simulink model "timertest"  (R2019a)
settings: Solver=VariableStepAuto  StartTime=0.0  StopTime=3600 * 24 * 60  RelTol=1e-3
undefined symbols (not defined in the file or in its folder): f
libraries: instrumentlib x2
settings Model: Creator=brandt  LastModifiedBy=brandt

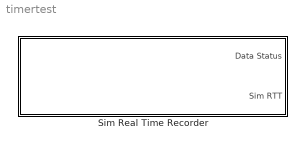
== system timertest ==
  Sim Real Time Recorder : Subsystem  AncestorBlock=gasLibrary/Sim Real Time Recorder

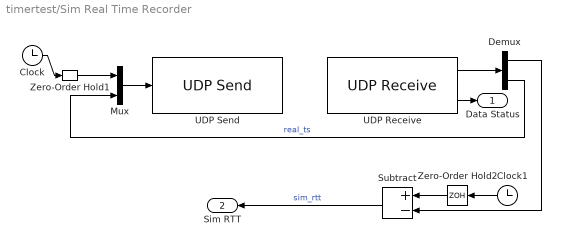
== system timertest/Sim Real Time Recorder ==
  Clock : Clock
  Clock1 : Clock
  Demux : Demux  Outputs=2
  Mux : Mux  Inputs=2
  Subtract : Sum  Inputs=+-
  UDP Receive : instrumentlib/UDP Receive  Priority=2  Host=localhost  Port=5001  LocalPort=6065  EnablePortSharing=off  GetLatestData=off  DataSize="[2  1]"  DataType=double  ASCIIFormatting=%f,  Terminator=LF  ByteOrder=BigEndian  EnableBlockingMode=off  Timeout=50  SampleTime=60  LocalAddress=localhost
      settings: SourceProductName=Instrument Control Toolbox
  UDP Send : instrumentlib/UDP Send  Priority=1  Host=localhost  Port=6068  LocalPort=-1  EnablePortSharing=off  ByteOrder=BigEndian  OutputDatagramPacketSize=24  EnableBlockingMode=on  LocalAddress=0.0.0.0
      settings: SourceProductName=Instrument Control Toolbox
  Zero-Order Hold1 : ZeroOrderHold  SampleTime=60
  Zero-Order Hold2 : ZeroOrderHold  SampleTime=60
  Data Status : Outport
  Sim RTT : Outport  Port=2
  wires:
  Clock1/1 -> Zero-Order Hold2/1
  Clock/1 -> Zero-Order Hold1/1
  Demux/1 -> Subtract/2
  UDP Receive/1 -> Demux/1
  Demux/2 -> Mux/2  "real_ts"
  UDP Receive/2 -> Data Status/1
  Mux/1 -> UDP Send/1
  Zero-Order Hold2/1 -> Subtract/1
  Zero-Order Hold1/1 -> Mux/1
  Subtract/1 -> Sim RTT/1  "sim_rtt"
